simulink model "smm_with_grf_tilting_2d"  (R2014b)
settings: Solver=FixedStepDiscrete  StartTime=0.0  StopTime=inf  FixedStep=sample_time  RelTol=1e-3
undefined symbols (not defined in the file or in its folder): A_lpf_dtau, A_lpf_leg_spring, alpha_apex, alpha_max, alpha_min, B1_lpf_dtau, B1_lpf_leg_spring, B2_lpf_dtau, B2_lpf_leg_spring, boom_mount_angle, boom_pelvis_offset_angle, c_energy, contact_threshold, control_start_time, d_y_boom_com_offset, d_y_boom_hip_offset, d_y_com, desired_torso_angle, dx_avg_desired, enable_torso_wave, fcut_contact, ff_energy_l, ff_energy_r, g, g_reduced, h_boom, HIP_MTR_MAX_CONT_TORQUE, i_robot, initial_com_height, initial_dx, j_leg, j_motor, j_rotor, j_segments, k0_virtual, k_placement, k_sea, kd_lateral, kd_motor, kd_torso, kp_lateral, kp_motor, kp_raibert, kp_torso, l0_leg, l0_min_flight_time, l0_virtual, l0_virtual_raibert, l_boom_projected, l_max, l_retract_delta, l_retract_swing_max, l_retract_swing_min, l_seg, l_yaw_center_to_pelvis, lambda1, lambda2, lateral_offset, lateral_target_angle_left, lateral_target_angle_right ... (+40)
libraries: simulink x24, slrtlib x4, simulink_extras x2
(part 2 of 4)

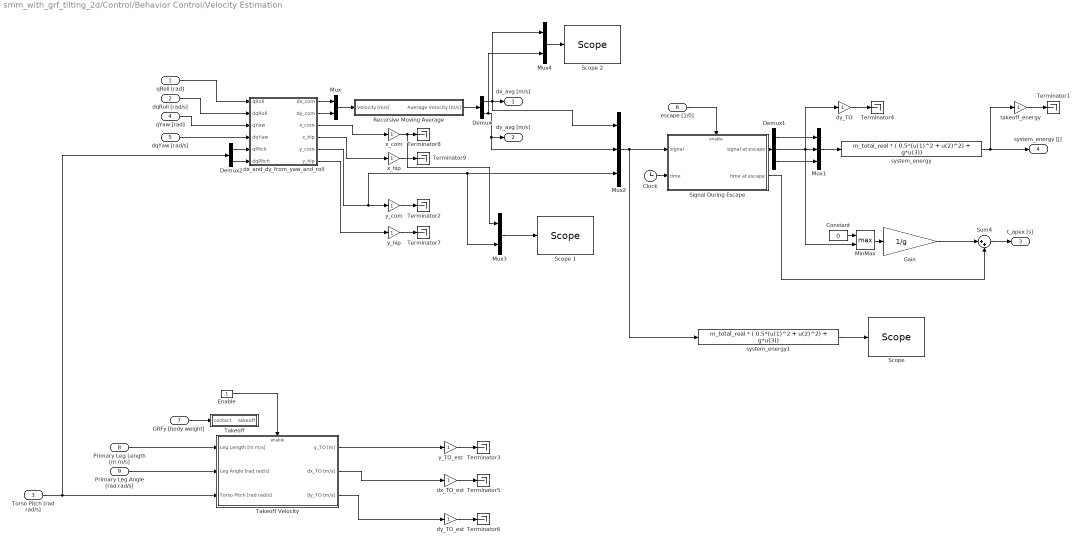
== system smm_with_grf_tilting_2d/Control/Behavior Control/Velocity Estimation ==
  qRoll [rad] : Inport
  dqRoll [rad/s] : Inport  Port=2
  Torso Pitch [rad rad/s] : Inport  Port=3
  qYaw [rad] : Inport  Port=4
  dqYaw [rad/s] : Inport  Port=5
  escape [1/0] : Inport  Port=6
  GRFy [body weight] : Inport  Port=7
  Primary Leg Length [m m/s] : Inport  Port=8
  Primary Leg Angle [rad rad/s] : Inport  Port=9
  Clock : Clock
  Constant : Constant  Value=0
  Demux : Demux  Outputs=2
  Demux1 : Demux  Outputs=3
  Demux2 : Demux  Outputs=2
  Enable : Constant  OutDataTypeStr=boolean
  Gain : Gain  Gain=1/g
  MinMax : MinMax  Function=max  Inputs=2
  Mux : Mux  Inputs=2
  Mux1 : Mux  Inputs=3
  Mux2 : Mux  Inputs=3
  Mux3 : Mux  Inputs=2
  Mux4 : Mux  Inputs=2
  Recursive Moving Average : Subsystem
  "Scope " : slrtlib/Displays and Logging/Scope   scopeno=2  scopetype=Host  autostart=on  viewmode=Graphical redraw  formatstr='%15.6f'  grid=on  ylimits=[0,0]  nosamples=4*250  noprepostsamples=0  interleave=4  triggermode=FreeRun  triggersignal=1  trigsignalfromport=off  triggerlevel=0.0  triggerslope=Either  triggerscope=1  triggersample=0  filename=data.dat  mode=Lazy  writesize=512  autorestart=off  dynamicfilemode=off  maxwritefilesize=512*1024^2
  Scope 1 : slrtlib/Displays and Logging/Scope   scopeno=1  scopetype=Host  autostart=on  viewmode=Graphical redraw  formatstr='%15.6f'  grid=on  ylimits=[0,0]  nosamples=4*250  noprepostsamples=0  interleave=4  triggermode=FreeRun  triggersignal=1  trigsignalfromport=off  triggerlevel=0.0  triggerslope=Either  triggerscope=1  triggersample=0  filename=data.dat  mode=Lazy  writesize=512  autorestart=off  dynamicfilemode=off  maxwritefilesize=512*1024^2
  Scope 2 : slrtlib/Displays and Logging/Scope   scopeno=3  scopetype=Host  autostart=on  viewmode=Graphical redraw  formatstr='%15.6f'  grid=on  ylimits=[0,0]  nosamples=4*250  noprepostsamples=0  interleave=4  triggermode=FreeRun  triggersignal=1  trigsignalfromport=off  triggerlevel=0.0  triggerslope=Either  triggerscope=1  triggersample=0  filename=data.dat  mode=Lazy  writesize=512  autorestart=off  dynamicfilemode=off  maxwritefilesize=512*1024^2
  Signal During Escape : Subsystem
  Sum4 : Sum  Inputs=|++
  Takeoff : Subsystem
  Takeoff Velocity : Subsystem
  Terminator{1..9} (9 alike) : Terminator
  dx_TO_est : Gain
  dx_and_dy_from_yaw_and_roll : MATLAB Function  TreatAsAtomicUnit=on
  dy_TO : Gain
  dy_TO_est : Gain
  system_energy : Fcn  Expr=m_total_real * ( 0.5*(u(1)^2 + u(2)^2) + g*u(3))
  system_energy1 : Fcn  Expr=m_total_real * ( 0.5*(u(1)^2 + u(2)^2) + g*u(3))
  takeoff_energy : Gain
  x_com : Gain
  x_hip : Gain
  y_TO_est : Gain
  y_com : Gain
  y_hip : Gain
  dx_avg [m/s] : Outport
  dy_avg [m/s] : Outport  Port=2
  t_apex [s] : Outport  Port=3
  system_energy [J] : Outport  Port=4
  wires:
  Gain/1 -> Sum4/1
  Enable/1 -> Takeoff Velocity/Enable
  dx_and_dy_from_yaw_and_roll/6(y_hip) -> y_hip/1
  y_hip/1 -> Terminator7/1
  Takeoff Velocity/3(dy_TO [m/s]) -> dy_TO_est/1
  dy_TO_est/1 -> Terminator6/1
  Takeoff Velocity/2(dx_TO [m/s]) -> dx_TO_est/1
  dx_TO_est/1 -> Terminator5/1
  y_TO_est/1 -> Terminator3/1
  Takeoff Velocity/1(y_TO [m]) -> y_TO_est/1
  y_com/1 -> Terminator2/1
  system_energy/1 -> takeoff_energy/1, system_energy [J]/1
  Clock/1 -> Signal During Escape/2(time)
  Demux1/3 -> Mux1/3
  Signal During Escape/2(time at escape) -> Sum4/2
  Signal During Escape/1(signal at escape) -> Demux1/1
  escape [1/0]/1 -> Signal During Escape/Enable
  takeoff_energy/1 -> Terminator1/1
  dy_TO/1 -> Terminator4/1
  Mux1/1 -> system_energy/1
  Demux1/1 -> Mux1/1
  Demux1/2 -> MinMax/2, dy_TO/1, Mux1/2
  Torso Pitch [rad rad/s]/1 -> Demux2/1, Takeoff Velocity/3(Torso Pitch [rad rad/s])
  Primary Leg Angle [rad rad/s]/1 -> Takeoff Velocity/2(Leg Angle [rad rad/s])
  Primary Leg Length [m m/s]/1 -> Takeoff Velocity/1(Leg Length [m m/s])
  Sum4/1 -> t_apex [s]/1
  Demux/2 -> Mux4/2, Mux2/2, dy_avg [m/s]/1
  Demux/1 -> Mux2/1, Mux4/1, dx_avg [m/s]/1
  Mux/1 -> Recursive Moving Average/1(Velocity [m/s])
  dx_and_dy_from_yaw_and_roll/2(dy_com) -> Mux/2
  GRFy [body weight]/1 -> Takeoff/1(contact)
  dx_and_dy_from_yaw_and_roll/1(dx_com) -> Mux/1
  Recursive Moving Average/1(Average Velocity [m/s]) -> Demux/1
  MinMax/1 -> Gain/1
  Constant/1 -> MinMax/1
  x_hip/1 -> Terminator9/1
  x_com/1 -> Mux3/1, Terminator8/1
  dx_and_dy_from_yaw_and_roll/3(x_com) -> x_com/1
  dx_and_dy_from_yaw_and_roll/4(x_hip) -> x_hip/1
  Demux2/1 -> dx_and_dy_from_yaw_and_roll/5(qPitch)
  Demux2/2 -> dx_and_dy_from_yaw_and_roll/6(dqPitch)
  qRoll [rad]/1 -> dx_and_dy_from_yaw_and_roll/1(qRoll)
  dqRoll [rad/s]/1 -> dx_and_dy_from_yaw_and_roll/2(dqRoll)
  qYaw [rad]/1 -> dx_and_dy_from_yaw_and_roll/3(qYaw)
  dqYaw [rad/s]/1 -> dx_and_dy_from_yaw_and_roll/4(dqYaw)
  Mux2/1 -> system_energy1/1, Signal During Escape/1(signal)
  system_energy1/1 -> "Scope "/1
  Mux3/1 -> Scope 1/1
  dx_and_dy_from_yaw_and_roll/5(y_com) -> Mux3/2, Mux2/3, y_com/1
  Mux4/1 -> Scope 2/1

== system smm_with_grf_tilting_2d/Control/Behavior Control/Virtual Spring Calculator ==
  "Stance Leg Angle [rad rad/s] " : Inport
  Stance Leg Length [m m/s] : Inport  Port=2
  Torso Angle [rad rad/s] : Inport  Port=3
  Demux : Demux  Outputs=2
  Demux1 : Demux  Outputs=2
  Demux2 : Demux  Outputs=2
  Mux3 : Mux  Inputs=2
  Mux4 : Mux  Inputs=2
  Virtual Spring Calculations : MATLAB Function  TreatAsAtomicUnit=on
  Spring Length [m m/s] : Outport
  Spring Alpha [rad rad/s] : Outport  Port=2  OutDataTypeStr=double  PortDimensions=2
  wires:
  Stance Leg Length [m m/s]/1 -> Demux1/1
  Mux3/1 -> Spring Length [m m/s]/1
  "Stance Leg Angle [rad rad/s] "/1 -> Demux2/1
  Torso Angle [rad rad/s]/1 -> Demux/1
  Demux/1 -> Virtual Spring Calculations/1(th)
  Demux/2 -> Virtual Spring Calculations/2(dth)
  Demux1/1 -> Virtual Spring Calculations/3(l)
  Demux2/1 -> Virtual Spring Calculations/5(phi)
  Demux2/2 -> Virtual Spring Calculations/6(dphi)
  Demux1/2 -> Virtual Spring Calculations/4(dl)
  Virtual Spring Calculations/1(alpha_v) -> Mux4/1
  Virtual Spring Calculations/2(dalpha_v) -> Mux4/2
  Virtual Spring Calculations/3(l_v) -> Mux3/1
  Virtual Spring Calculations/4(dl_v) -> Mux3/2
  Mux4/1 -> Spring Alpha [rad rad/s]/1

== system smm_with_grf_tilting_2d/Control/Behavior Control/dtau_des ==
  x : Inport
  Gain1 : Gain  Gain=1/sample_time
  difference : simulink/Discrete/Difference  ICPrevInput=0.0  InputProcessing=Inherited  OutMin=[]  OutMax=[]  OutDataType=fixdt(1, 16)  OutScaling=2^-10  DoSatur=off
  two_pole_filter : DiscreteTransferFcn  Numerator=[A_lpf_dtau 0 0]  Denominator=[1 B1_lpf_dtau B2_lpf_dtau]  SampleTime=sample_time
  dx/dt : Outport
  wires:
  two_pole_filter/1 -> dx/dt/1
  x/1 -> Gain1/1
  difference/1 -> two_pole_filter/1
  Gain1/1 -> difference/1

== system smm_with_grf_tilting_2d/Control/Behavior Control/Contact Estimation/Contact Time ==
  Enable : EnablePort  StatesWhenEnabling=reset  ShowOutputPort=on
  Constant : Constant
  Discrete-Time Integrator : DiscreteIntegrator  IntegratorMethod=Accumulation: Forward Euler  gainval=sample_time  ExternalReset=rising  SampleTime=sample_time
  ts [s] : Outport  InitialOutput=[0]
  wires:
  Discrete-Time Integrator/1 -> ts [s]/1
  Enable/1 -> Discrete-Time Integrator/2
  Constant/1 -> Discrete-Time Integrator/1

== system smm_with_grf_tilting_2d/Control/Behavior Control/Contact Estimation/Last Contact Time ==
  ts [s] : Inport
  Trigger : TriggerPort  TriggerType=falling  PortDimensions=1
  Ts [s] : Outport  InitialOutput=[0]
  wires:
  ts [s]/1 -> Ts [s]/1

== system smm_with_grf_tilting_2d/Control/Behavior Control/Contact Estimation/Leg Force Measurements ==
  q : Inport
  w right/left [m m] : Inport  Port=2
  Demux : Demux  Outputs=2
  Divide1 : Product  Inputs=*/
  Divide2 : Product  Inputs=*/
  Spring Stiffness3 : Gain  Gain=k_sea(1)
  Spring Stiffness4 : Gain  Gain=k_sea(3)
  Spring Stiffness5 : Gain  Gain=k_sea(2)
  Spring Stiffness6 : Gain  Gain=k_sea(4)
  Sum{1..6} (6 alike) : Sum  Inputs=-+|
  backGearL : Selector  InputPortWidth=13  Indices=[6]
  backGearR : Selector  InputPortWidth=13  Indices=[2]
  backJointL : Selector  InputPortWidth=13  Indices=[5]
  backJointR : Selector  InputPortWidth=13  Indices=[1]
  frontGearL : Selector  InputPortWidth=13  Indices=[8]
  frontGearR : Selector  InputPortWidth=13  Indices=[4]
  frontJointL : Selector  InputPortWidth=13  Indices=[7]
  frontJointR : Selector  InputPortWidth=13  Indices=[3]
  Right Leg Force [N] : Outport
  Left Leg Force [N] : Outport  Port=2
  wires:
  Sum3/1 -> Spring Stiffness6/1
  Sum2/1 -> Spring Stiffness4/1
  backJointL/1 -> Sum2/1
  frontGearL/1 -> Sum3/2
  frontJointL/1 -> Sum3/1
  backGearL/1 -> Sum2/2
  Sum6/1 -> Spring Stiffness3/1
  Sum1/1 -> Spring Stiffness5/1
  backJointR/1 -> Sum6/1
  frontGearR/1 -> Sum1/2
  frontJointR/1 -> Sum1/1
  backGearR/1 -> Sum6/2
  q/1 -> backGearR/1, backJointL/1, backGearL/1, frontJointR/1, frontGearR/1, frontJointL/1, frontGearL/1, backJointR/1
  Spring Stiffness3/1 -> Sum4/1
  Spring Stiffness5/1 -> Sum4/2
  Spring Stiffness6/1 -> Sum5/2
  Spring Stiffness4/1 -> Sum5/1
  Sum4/1 -> Divide1/1
  Sum5/1 -> Divide2/1
  w right/left [m m]/1 -> Demux/1
  Demux/1 -> Divide1/2
  Demux/2 -> Divide2/2
  Divide1/1 -> Right Leg Force [N]/1
  Divide2/1 -> Left Leg Force [N]/1

== system smm_with_grf_tilting_2d/Control/Behavior Control/Contact Estimation/Vertical Spring Force ==
  theta [rad] : Inport
  phi [rad] : Inport  Port=2
  Force [N] : Inport  Port=3
  Gain : Gain  Gain=-1
  Product : Product
  Sum : Sum  Inputs=++|
  Trigonometric Function : Trigonometry  Operator=cos
  Vertical Force [N] : Outport
  wires:
  Gain/1 -> Vertical Force [N]/1
  Sum/1 -> Trigonometric Function/1
  Product/1 -> Gain/1
  Trigonometric Function/1 -> Product/2
  theta [rad]/1 -> Sum/1
  phi [rad]/1 -> Sum/2
  Force [N]/1 -> Product/1

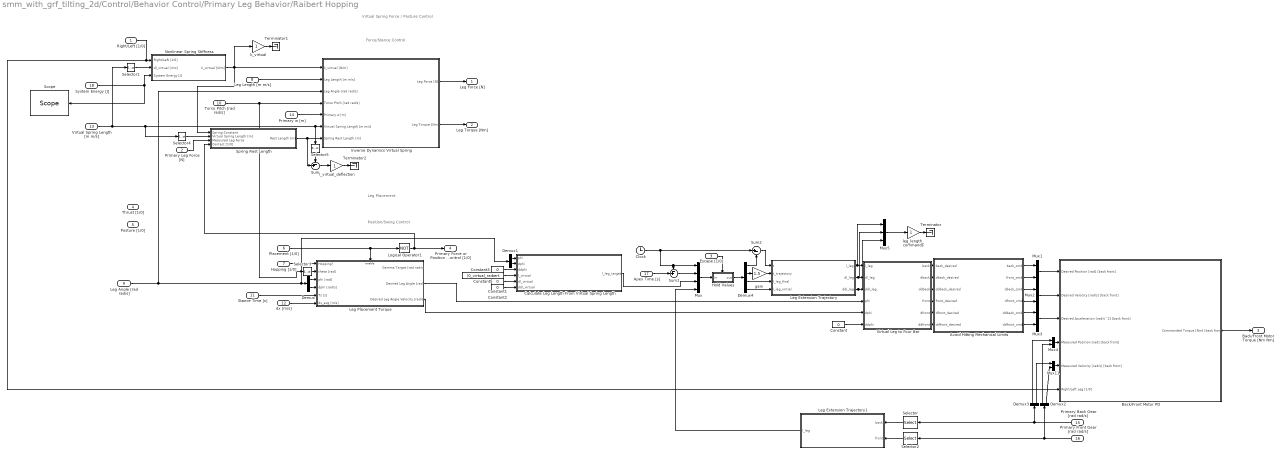
== system smm_with_grf_tilting_2d/Control/Behavior Control/Primary Leg Behavior/Raibert Hopping ==
  note: Leg Placement
  note: Virtual Spring Force / Posture Control
  note: Force/Stance Control
  note: Position/Swing Control
  Right/Left [1/0] : Inport
  Primary Leg Force [N] : Inport  Port=2
  Escape [1/0] : Inport  Port=3
  Thrust [1/0] : Inport  Port=4
  Posture [1/0] : Inport  Port=5
  Placement [1/0] : Inport  Port=6
  Hopping [1/0] : Inport  Port=7
  Leg Length [m m/s] : Inport  Port=8
  Leg Angle [rad rad/s] : Inport  Port=9
  Torso Pitch [rad rad/s] : Inport  Port=10
  Stance Time [s] : Inport  Port=11
  dx [m/s] : Inport  Port=12
  Virtual Spring Length [m m/s] : Inport  Port=13
  Primary w [m] : Inport  Port=14
  Primary Back Gear [rad rad/s] : Inport  Port=15
  Primary Front Gear [rad rad/s] : Inport  Port=16
  Apex Time [s] : Inport  Port=17
  System Energy [J] : Inport  Port=18
  Avoid Hitting Mechanical Limits : MATLAB Function  TreatAsAtomicUnit=on
  Back/Front Motor PD : Subsystem
  Calculate Leg Length From Virtual Spring Length : MATLAB Function  TreatAsAtomicUnit=on
  Clock : Clock
  Constant{,1..3} (4 alike) : Constant  Value=0
  Constant5 : Constant  Value=l0_virtual_raibert
  Demux{,1..3} (4 alike) : Demux  Outputs=2
  Demux4 : Demux
  Hold Values : Subsystem
  Inverse Dynamics Virtual Spring : Subsystem
  Leg Extension Trajectory : MATLAB Function  TreatAsAtomicUnit=on
  Leg Extension Trajectory1 : MATLAB Function  TreatAsAtomicUnit=on
  Leg Placement Torque : Subsystem
  Logical Operator1 : Logic  Operator=NOT  AllPortsSameDT=off  OutDataTypeStr=boolean
  Mux : Mux
  Mux{1..4,11} (5 alike) : Mux  Inputs=2
  Mux5 : Mux  Inputs=3
  Nonlinear Spring Stiffness : Subsystem
  "Scope " : slrtlib/Displays and Logging/Scope   scopeno=5  scopetype=Host  autostart=on  viewmode=Graphical redraw  formatstr='%15.6f'  grid=on  ylimits=[0,0]  nosamples=4*250  noprepostsamples=0  interleave=4  triggermode=FreeRun  triggersignal=1  trigsignalfromport=off  triggerlevel=0.0  triggerslope=Either  triggerscope=1  triggersample=0  filename=data.dat  mode=Lazy  writesize=512  autorestart=off  dynamicfilemode=off  maxwritefilesize=512*1024^2
  Selector{,2..5} (5 alike) : Selector  InputPortWidth=2  Indices=[1]
  Selector1 : Selector  InputPortWidth=2  Indices=[2]
  Spring Rest Length : Subsystem
  Sum : Sum  Inputs=-+|
  Sum1 : Sum  Inputs=-+|
  Sum2 : Sum  Inputs=|+-
  Terminator : Terminator
  Terminator1 : Terminator
  Terminator2 : Terminator
  Virtual Leg to Four Bar : MATLAB Function  TreatAsAtomicUnit=on
  gain : Gain  Gain=1.5
  k_virtual : Gain
  l_virtual_deflection : Gain
  leg_length_commands : Gain
  Leg Force [N] : Outport
  Leg Torque [Nm] : Outport  Port=2
  Back/Front Motor Torque [Nm Nm] : Outport  Port=3
  Primary Force or Position Control [1/0] : Outport  Port=4  OutDataTypeStr=boolean
  wires:
  Nonlinear Spring Stiffness/1(k_virtual [N/m]) -> Spring Rest Length/1(Spring Constant), k_virtual/1, Inverse Dynamics Virtual Spring/1(k_virtual [N/m])
  Selector1/1 -> Nonlinear Spring Stiffness/2(dl_virtual [m/s])
  Demux/1 -> Leg Placement Torque/3(phi [rad])
  Demux/2 -> Leg Placement Torque/4(dphi [rad/s])
  Hopping [1/0]/1 -> Leg Placement Torque/1(Hopping?)
  Placement [1/0]/1 -> Leg Placement Torque/Enable, Logical Operator1/1
  Selector3/1 -> Leg Placement Torque/2(theta [rad])
  Torso Pitch [rad rad/s]/1 -> Selector3/1, Inverse Dynamics Virtual Spring/4(Torso Pitch [rad rad/s])
  Leg Length [m m/s]/1 -> Inverse Dynamics Virtual Spring/2(Leg Length [m m/s])
  dx [m/s]/1 -> Leg Placement Torque/6(dx_avg [m/s])
  Stance Time [s]/1 -> Leg Placement Torque/5(Ts [s])
  Virtual Spring Length [m m/s]/1 -> Inverse Dynamics Virtual Spring/6(Virtual Spring Length [m m/s]), Selector5/1, Selector4/1, Selector1/1
  Leg Angle [rad rad/s]/1 -> Demux1/1, Demux/1, Inverse Dynamics Virtual Spring/3(Leg Angle [rad rad/s])
  Primary w [m]/1 -> Inverse Dynamics Virtual Spring/5(Primary w [m])
  Inverse Dynamics Virtual Spring/2(Leg Torque [Nm]) -> Leg Torque [Nm]/1
  Inverse Dynamics Virtual Spring/1(Leg Force [N]) -> Leg Force [N]/1
  Virtual Leg to Four Bar/1(back) -> Avoid Hitting Mechanical Limits/1(back_desired)
  Virtual Leg to Four Bar/2(dback) -> Avoid Hitting Mechanical Limits/2(dback_desired)
  Virtual Leg to Four Bar/3(ddback) -> Avoid Hitting Mechanical Limits/3(ddback_desired)
  Virtual Leg to Four Bar/4(front) -> Avoid Hitting Mechanical Limits/4(front_desired)
  Virtual Leg to Four Bar/5(dfront) -> Avoid Hitting Mechanical Limits/5(dfront_desired)
  Virtual Leg to Four Bar/6(ddfront) -> Avoid Hitting Mechanical Limits/6(ddfront_desired)
  Mux11/1 -> Back/Front Motor PD/5(Measured Velocity [rad/s] [back front])
  Demux2/2 -> Mux11/2
  Mux4/1 -> Back/Front Motor PD/4(Measured Position [rad] [back front])
  Mux1/1 -> Back/Front Motor PD/1(Desired Position [rad] [back front])
  Demux3/2 -> Mux11/1
  Demux3/1 -> Mux4/1
  Avoid Hitting Mechanical Limits/2(front_cmd) -> Mux1/2
  Avoid Hitting Mechanical Limits/1(back_cmd) -> Mux1/1
  Demux2/1 -> Mux4/2
  Avoid Hitting Mechanical Limits/3(dback_cmd) -> Mux2/1
  Avoid Hitting Mechanical Limits/4(dfront_cmd) -> Mux2/2
  Avoid Hitting Mechanical Limits/5(ddback_cmd) -> Mux3/1
  Avoid Hitting Mechanical Limits/6(ddfront_cmd) -> Mux3/2
  Mux2/1 -> Back/Front Motor PD/2(Desired Velocity [rad/s] [back front])
  Mux3/1 -> Back/Front Motor PD/3(Desired Acceleration [rad/s^2] [back front])
  Logical Operator1/1 -> Spring Rest Length/4(Contact [1/0]), Primary Force or Position Control [1/0]/1
  Back/Front Motor PD/1(Commanded Torque [Nm] [back front]) -> Back/Front Motor Torque [Nm Nm]/1
  Primary Back Gear [rad rad/s]/1 -> Demux3/1, Selector/1
  Primary Front Gear [rad rad/s]/1 -> Selector2/1, Demux2/1
  Constant/1 -> Virtual Leg to Four Bar/6(ddphi)
  Leg Placement Torque/2(Desired Leg Angle [rad]) -> Virtual Leg to Four Bar/4(phi)
  Leg Placement Torque/3(Desired Leg Angle Velocity [rad/s]) -> Virtual Leg to Four Bar/5(dphi)
  Constant5/1 -> Calculate Leg Length From Virtual Spring Length/4(l_virtual)
  Constant1/1 -> Calculate Leg Length From Virtual Spring Length/5(dl_virtual)
  Constant2/1 -> Calculate Leg Length From Virtual Spring Length/6(ddl_virtual)
  Constant3/1 -> Calculate Leg Length From Virtual Spring Length/3(ddphi)
  Demux1/1 -> Calculate Leg Length From Virtual Spring Length/1(phi)
  Demux1/2 -> Calculate Leg Length From Virtual Spring Length/2(dphi)
  Leg Extension Trajectory/1(l_leg) -> Mux5/1, Virtual Leg to Four Bar/1(l_leg)
  Leg Extension Trajectory/3(ddl_leg) -> Mux5/3, Virtual Leg to Four Bar/3(ddl_leg)
  Apex Time [s]/1 -> Sum1/2
  Clock/1 -> Sum1/1, Mux/1, Sum2/1
  Sum2/1 -> Leg Extension Trajectory/1(t)
  Mux5/1 -> leg_length_commands/1
  Leg Extension Trajectory/2(dl_leg) -> Mux5/2, Virtual Leg to Four Bar/2(dl_leg)
  leg_length_commands/1 -> Terminator/1
  Demux4/2 -> gain/1
  Sum1/1 -> Mux/2
  Calculate Leg Length From Virtual Spring Length/1(l_leg_target) -> Mux/3
  Demux4/4 -> Leg Extension Trajectory/4(l_leg_initial)
  Demux4/3 -> Leg Extension Trajectory/3(l_leg_final)
  Demux4/1 -> Sum2/2
  Selector/1 -> Leg Extension Trajectory1/1(back)
  Selector2/1 -> Leg Extension Trajectory1/2(front)
  Right/Left [1/0]/1 -> Back/Front Motor PD/6(Right/Left Leg [1/0]), Nonlinear Spring Stiffness/1(Right/Left [1/0])
  Hold Values/1(out) -> Demux4/1
  Mux/1 -> Hold Values/1(in)
  gain/1 -> Leg Extension Trajectory/2(t_trajectory)
  Escape [1/0]/1 -> Hold Values/Trigger
  Leg Extension Trajectory1/1(l_leg) -> Mux/4
  k_virtual/1 -> Terminator1/1
  l_virtual_deflection/1 -> Terminator2/1
  Sum/1 -> l_virtual_deflection/1
  Selector5/1 -> Sum/1
  Spring Rest Length/1(Rest Length [m]) -> Sum/2, Inverse Dynamics Virtual Spring/7(Spring Rest Length [m])
  Selector4/1 -> Spring Rest Length/2(Virtual Spring Length [m])
  Primary Leg Force [N]/1 -> Spring Rest Length/3(Measured Leg Force)
  System Energy [J]/1 -> Nonlinear Spring Stiffness/3(System Energy [J]), "Scope "/1

== system smm_with_grf_tilting_2d/Control/Behavior Control/Primary Leg Behavior/SMM 01 ==
  note: Stance
  note: Swing
  Right/Left [1/0] : Inport
  Escape [1/0] : Inport  Port=2
  Posture [1/0] : Inport  Port=3
  Placement [1/0] : Inport  Port=4
  Primary Leg Angle [rad rad/s] : Inport  Port=5
  Primary Leg Length [m m/s] : Inport  Port=6
  Torso Pitch [rad rad/s] : Inport  Port=7
  Virtual Spring Length [m m/s] : Inport  Port=8
  Apex Time [s] : Inport  Port=9
  System Energy [J] : Inport  Port=10
  Primary Back Gear [rad rad/s] : Inport  Port=11
  Primary Front Gear [rad rad/s] : Inport  Port=12
  Primary w [m] : Inport  Port=13
  Logical Operator : Logic  Operator=NOT  AllPortsSameDT=off  OutDataTypeStr=boolean
  Primary Stance Phase : Subsystem
  Primary Swing Phase : Subsystem
  Leg Force [Nm] : Outport
  Leg Torque [Nm] : Outport  Port=2
  Back/Front Motor Torque [Nm Nm] : Outport  Port=3
  Primary Force or Position Control [1/0] : Outport  Port=4  OutDataTypeStr=boolean
  wires:
  Primary w [m]/1 -> Primary Stance Phase/7(Primary w [m])
  Logical Operator/1 -> Primary Force or Position Control [1/0]/1
  Primary Stance Phase/2(Leg Force Command [Nm]) -> Leg Force [Nm]/1
  Primary Stance Phase/1(Leg Torque Command [Nm]) -> Leg Torque [Nm]/1
  Escape [1/0]/1 -> Primary Swing Phase/1(Escape [1/0])
  Virtual Spring Length [m m/s]/1 -> Primary Stance Phase/6(Virtual Spring Length [m m/s])
  System Energy [J]/1 -> Primary Stance Phase/5(System Energy [J])
  Posture [1/0]/1 -> Primary Stance Phase/3(Enable Posture Control [1/0])
  Primary Leg Angle [rad rad/s]/1 -> Primary Swing Phase/3(Primary Leg Angle [rad rad/s]), Primary Stance Phase/8(Primary Leg Angle [rad rad/s])
  Primary Swing Phase/1(Back/Front Motor Torque Command [Nm Nm]) -> Back/Front Motor Torque [Nm Nm]/1
  Primary Front Gear [rad rad/s]/1 -> Primary Swing Phase/7(Primary Front Gear [rad rad/s])
  Primary Back Gear [rad rad/s]/1 -> Primary Swing Phase/6(Primary Back Gear [rad rad/s])
  Apex Time [s]/1 -> Primary Swing Phase/5(Time of Apex [s])
  Placement [1/0]/1 -> Logical Operator/1
  Right/Left [1/0]/1 -> Primary Stance Phase/4(Right/Left Primary [1/0]), Primary Swing Phase/8(Right/Left Primary [1/0])
  Primary Leg Length [m m/s]/1 -> Primary Swing Phase/2(Primary Leg Length [m m/s]), Primary Stance Phase/1(Primary Leg Length [m m/s])
  Torso Pitch [rad rad/s]/1 -> Primary Swing Phase/4(Torso Pitch [rad rad/s]), Primary Stance Phase/2(Torso Pitch [rad rad/s])

== system smm_with_grf_tilting_2d/Control/Behavior Control/Secondary Leg Behavior/Back//Front Motor PD ==
  Desired Position [rad] [back front] : Inport
  Desired Velocity [rad/s] [back front] : Inport  Port=2
  Desired Acceleration [rad/s^2] [back front] : Inport  Port=3
  Measured Position [rad] [back front] : Inport  Port=4
  Measured Velocity [rad/s] [back front] : Inport  Port=5
  Right/Left Leg [1/0] : Inport  Port=6
  Friction Compensation : Subsystem
  Product : Product
  Sum1 : Sum  Inputs=|++
  Sum2 : Sum  Inputs=|++
  Sum7 : Sum  Inputs=|+-
  Sum8 : Sum  Inputs=|+-
  Sum9 : Sum
  Switch : Switch  Criteria=u2 ~= 0
  kd : Gain  Gain=kd_motor
  kp : Gain  Gain=kp_motor
  left_inertias : Constant  Value=j_segments(3:4)
  reflected inertia : Constant  Value=j_motor
  right_inertias : Constant  Value=j_segments(1:2)
  Commanded Torque [Nm] [back front] : Outport
  wires:
  kp/1 -> Sum9/1
  Sum7/1 -> kp/1
  Measured Position [rad] [back front]/1 -> Sum7/2
  Sum9/1 -> Sum1/1
  Sum8/1 -> kd/1
  Desired Position [rad] [back front]/1 -> Sum7/1
  kd/1 -> Sum9/2
  Measured Velocity [rad/s] [back front]/1 -> Sum8/2
  Sum1/1 -> Sum2/1
  Desired Acceleration [rad/s^2] [back front]/1 -> Product/1
  Product/1 -> Sum1/2
  Right/Left Leg [1/0]/1 -> Friction Compensation/1(Right/Left [1/0]), Switch/2
  right_inertias/1 -> Switch/1
  left_inertias/1 -> Switch/3
  Sum2/1 -> Commanded Torque [Nm] [back front]/1
  Desired Velocity [rad/s] [back front]/1 -> Friction Compensation/2(Commanded Velocity [rad/s] [back front]), Sum8/1
  reflected inertia/1 -> Product/2

== system smm_with_grf_tilting_2d/Control/Behavior Control/Velocity Estimation/Recursive Moving Average ==
  Velocity [m/s] : Inport
  Delay : Delay  DelayLength=velocity_avg_samples  InitialCondition=0  UseCircularBuffer=on  SampleTime=sample_time
  Gain : Gain  Gain=1/velocity_avg_samples
  Sum : Sum  Inputs=-++
  Unit Delay : UnitDelay  SampleTime=sample_time
  Average Velocity [m/s] : Outport
  wires:
  Unit Delay/1 -> Sum/3
  Gain/1 -> Average Velocity [m/s]/1
  Delay/1 -> Sum/1
  Sum/1 -> Gain/1, Unit Delay/1
  Velocity [m/s]/1 -> Sum/2, Delay/1

== system smm_with_grf_tilting_2d/Control/Behavior Control/Velocity Estimation/Signal During Escape ==
  signal : Inport
  time : Inport  Port=2
  Enable : EnablePort
  signal at escape : Outport  InitialOutput=[0 0 y_com_desired-0.1182]
  time at escape : Outport  Port=2
  wires:
  time/1 -> time at escape/1
  signal/1 -> signal at escape/1

== system smm_with_grf_tilting_2d/Control/Behavior Control/Velocity Estimation/Takeoff ==
  contact : Inport
  Compare To Constant : simulink/Logic and Bit Operations/Compare To Constant  relop=<=  const=TO_threshold  OutDataTypeStr=boolean
  Compare To Constant1 : simulink/Logic and Bit Operations/Compare To Constant  relop=>  const=TO_threshold  OutDataTypeStr=boolean
  Logical Operator : Logic  AllPortsSameDT=off  OutDataTypeStr=boolean
  Unit Delay1 : UnitDelay  SampleTime=sample_time
  takeoff : Outport
  wires:
  Unit Delay1/1 -> Compare To Constant1/1
  Logical Operator/1 -> takeoff/1
  contact/1 -> Unit Delay1/1, Compare To Constant/1
  Compare To Constant/1 -> Logical Operator/2
  Compare To Constant1/1 -> Logical Operator/1

== system smm_with_grf_tilting_2d/Control/Behavior Control/Velocity Estimation/Takeoff Velocity ==
  Leg Length [m m/s] : Inport
  Leg Angle [rad rad/s] : Inport  Port=2
  Torso Pitch [rad rad/s] : Inport  Port=3
  Enable : EnablePort
  Demux2 : Demux  Outputs=2
  Demux3 : Demux  Outputs=2
  Demux4 : Demux  Outputs=2
  vertical_velocity : MATLAB Function  TreatAsAtomicUnit=on
  y_TO [m] : Outport  InitialOutput=[initial_com_height]
  dx_TO [m/s] : Outport  Port=2  InitialOutput=[initial_dx]
  dy_TO [m/s] : Outport  Port=3  InitialOutput=[0]
  wires:
  vertical_velocity/3(dy) -> dy_TO [m/s]/1
  vertical_velocity/2(dx) -> dx_TO [m/s]/1
  vertical_velocity/1(y) -> y_TO [m]/1
  Demux2/2 -> vertical_velocity/2(dl)
  Demux4/2 -> vertical_velocity/6(dqPitch)
  Leg Angle [rad rad/s]/1 -> Demux3/1
  Demux3/1 -> vertical_velocity/3(phi)
  Demux3/2 -> vertical_velocity/4(dphi)
  Torso Pitch [rad rad/s]/1 -> Demux4/1
  Demux4/1 -> vertical_velocity/5(qPitch)
  Leg Length [m m/s]/1 -> Demux2/1
  Demux2/1 -> vertical_velocity/1(l)

== system smm_with_grf_tilting_2d/Control/Behavior Control/Primary Leg Behavior/Raibert Hopping/Back//Front Motor PD ==
  Desired Position [rad] [back front] : Inport
  Desired Velocity [rad/s] [back front] : Inport  Port=2
  Desired Acceleration [rad/s^2] [back front] : Inport  Port=3
  Measured Position [rad] [back front] : Inport  Port=4
  Measured Velocity [rad/s] [back front] : Inport  Port=5
  Right/Left Leg [1/0] : Inport  Port=6
  Friction Compensation : Subsystem
  Product : Product
  Sum1 : Sum  Inputs=|++
  Sum2 : Sum  Inputs=|++
  Sum7 : Sum  Inputs=|+-
  Sum8 : Sum  Inputs=|+-
  Sum9 : Sum
  kd : Gain  Gain=kd_motor
  kp : Gain  Gain=kp_motor
  reflected inertia : Constant  Value=j_motor
  Commanded Torque [Nm] [back front] : Outport
  wires:
  kp/1 -> Sum9/1
  Sum7/1 -> kp/1
  Measured Position [rad] [back front]/1 -> Sum7/2
  Sum9/1 -> Sum1/1
  Sum8/1 -> kd/1
  Desired Position [rad] [back front]/1 -> Sum7/1
  kd/1 -> Sum9/2
  Measured Velocity [rad/s] [back front]/1 -> Sum8/2
  Sum1/1 -> Sum2/1
  Desired Acceleration [rad/s^2] [back front]/1 -> Product/1
  Product/1 -> Sum1/2
  Right/Left Leg [1/0]/1 -> Friction Compensation/1(Right/Left [1/0])
  Sum2/1 -> Commanded Torque [Nm] [back front]/1
  Desired Velocity [rad/s] [back front]/1 -> Friction Compensation/2(Commanded Velocity [rad/s] [back front]), Sum8/1
  reflected inertia/1 -> Product/2
  Friction Compensation/1(Friction Compensation [Nm]) -> Sum2/2

== system smm_with_grf_tilting_2d/Control/Behavior Control/Primary Leg Behavior/Raibert Hopping/Hold Values ==
  in : Inport
  Trigger : TriggerPort  ShowOutputPort=on  PortDimensions=1
  Subsystem : Subsystem
  out : Outport
  wires:
  in/1 -> Subsystem/1(in)
  Subsystem/1(out) -> out/1
  Trigger/1 -> Subsystem/Enable

== system smm_with_grf_tilting_2d/Control/Behavior Control/Primary Leg Behavior/Raibert Hopping/Inverse Dynamics Virtual Spring ==
  k_virtual [N/m] : Inport
  Leg Length [m m/s] : Inport  Port=2
  Leg Angle [rad rad/s] : Inport  Port=3
  Torso Pitch [rad rad/s] : Inport  Port=4
  Primary w [m] : Inport  Port=5
  Virtual Spring Length [m m/s] : Inport  Port=6
  Spring Rest Length [m] : Inport  Port=7
  Angle Sine Wave : Subsystem  Commented=on
  Constant1 : Constant  Commented=on  Value=enable_torso_wave
  Constant2 : Constant  Value=0
  Constant3 : Constant  Value=desired_torso_angle
  Demux5 : Demux  Outputs=2
  GRF_angle : Gain
  GRFx_target : Gain
  GRFy_target : Gain
  Leg Force-Torque Distribution : Subsystem
  Spring Torques : Selector  InputPortWidth=7  Indices=[6 7]
  Terminator : Terminator
  Terminator1 : Terminator
  Terminator2 : Terminator
  target_GRF_inverse_dynamics : MATLAB Function  TreatAsAtomicUnit=on
  Leg Force [N] : Outport
  Leg Torque [Nm] : Outport  Port=2
  wires:
  Leg Force-Torque Distribution/1(Leg Force [N]) -> Leg Force [N]/1
  GRF_angle/1 -> Terminator2/1
  GRFy_target/1 -> Terminator1/1
  GRFx_target/1 -> Terminator/1
  Leg Angle [rad rad/s]/1 -> target_GRF_inverse_dynamics/4(phi)
  Torso Pitch [rad rad/s]/1 -> target_GRF_inverse_dynamics/3(theta)
  target_GRF_inverse_dynamics/4(GRF_angle) -> GRF_angle/1
  target_GRF_inverse_dynamics/3(GRFy) -> GRFy_target/1
  target_GRF_inverse_dynamics/2(GRFx) -> GRFx_target/1
  Leg Force-Torque Distribution/2(Leg Torque [Nm]) -> Leg Torque [Nm]/1
  Primary w [m]/1 -> target_GRF_inverse_dynamics/6(w), Leg Force-Torque Distribution/3(w [m])
  Spring Torques/1 -> Demux5/1
  Demux5/1 -> Leg Force-Torque Distribution/1(Front Spring Torque [Nm])
  Demux5/2 -> Leg Force-Torque Distribution/2(Back Spring Torque [Nm])
  target_GRF_inverse_dynamics/1(z) -> Spring Torques/1
  Constant2/1 -> target_GRF_inverse_dynamics/8(tau_rotor_b), target_GRF_inverse_dynamics/7(tau_rotor_f)
  Leg Length [m m/s]/1 -> target_GRF_inverse_dynamics/5(l_leg)
  k_virtual [N/m]/1 -> target_GRF_inverse_dynamics/1(k_virtual)
  Virtual Spring Length [m m/s]/1 -> target_GRF_inverse_dynamics/2(l_virtual)
  Constant1/1 -> Angle Sine Wave/Enable
  Spring Rest Length [m]/1 -> target_GRF_inverse_dynamics/9(l_virtual_rest)
  Constant3/1 -> target_GRF_inverse_dynamics/10(desired_torso_angle)

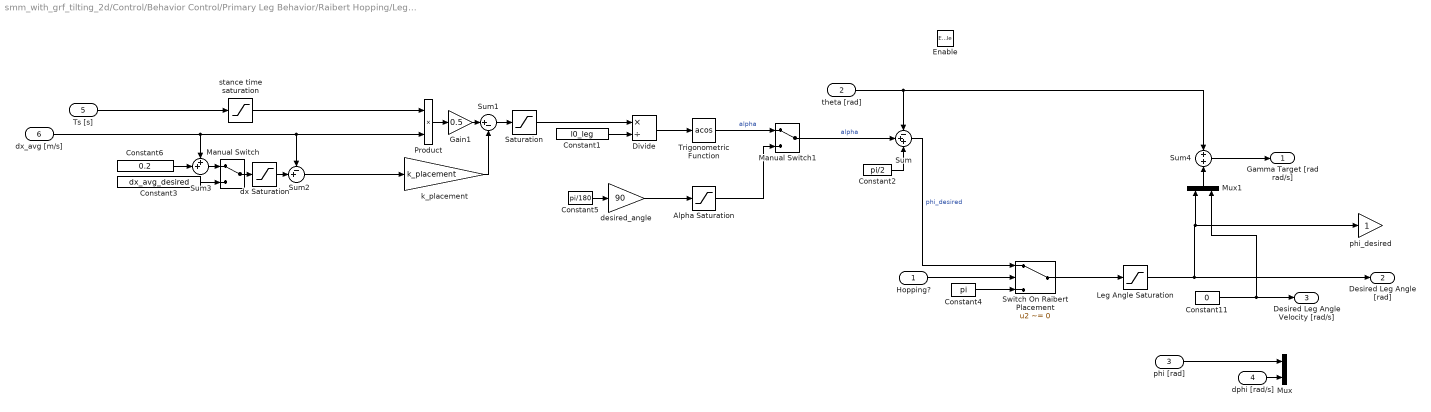
== system smm_with_grf_tilting_2d/Control/Behavior Control/Primary Leg Behavior/Raibert Hopping/Leg Placement Torque ==
  Hopping? : Inport
  theta [rad] : Inport  Port=2
  phi [rad] : Inport  Port=3
  dphi [rad/s] : Inport  Port=4
  Ts [s] : Inport  Port=5
  dx_avg [m/s] : Inport  Port=6
  Enable : EnablePort  StatesWhenEnabling=reset
  Alpha Saturation : Saturate  UpperLimit=alpha_max  LowerLimit=alpha_min
      settings: AttributesFormatString=Hi: %<UpperLimit>\nLo: %<LowerLimit>
  Constant1 : Constant  Value=l0_leg
  Constant11 : Constant  Value=0
  Constant2 : Constant  Value=pi/2
  Constant3 : Constant  Value=dx_avg_desired
  Constant4 : Constant  Value=pi
  Constant5 : Constant  Value=pi/180
  Constant6 : Constant  Value=0.2
  Divide : Product  Inputs=*/
  Gain1 : Gain  Gain=0.5
  Leg Angle Saturation : Saturate  UpperLimit=max_leg_angle  LowerLimit=min_leg_angle
      settings: AttributesFormatString=Hi: %<UpperLimit>\nLo: %<LowerLimit>
  Manual Switch : ManualSwitch
  Manual Switch1 : ManualSwitch
  Mux : Mux  Inputs=2
  Mux1 : Mux  Inputs=2
  Product : Product
  Saturation : Saturate  UpperLimit=x_limit  LowerLimit=-x_limit
      settings: AttributesFormatString=Hi: %<UpperLimit>\nLo: %<LowerLimit>
  Sum : Sum  Inputs=-++
  Sum1 : Sum  Inputs=|+-
  Sum2 : Sum  Inputs=-+|
  Sum3 : Sum  Inputs=++|
  Sum4 : Sum  Inputs=+|+
  Switch On Raibert Placement : Switch  Criteria=u2 ~= 0
  Trigonometric Function : Trigonometry  Operator=acos
  desired_angle : Gain  Gain=90
  dx Saturation : Saturate  UpperLimit=dx_avg_desired  LowerLimit=0
      settings: AttributesFormatString=Hi: %<UpperLimit>\nLo: %<LowerLimit>
  k_placement : Gain  Gain=k_placement
  phi_desired : Gain
  stance time saturation : Saturate  UpperLimit=1  LowerLimit=0
      settings: AttributesFormatString=Hi: %<UpperLimit>\nLo: %<LowerLimit>
  Gamma Target [rad rad/s] : Outport  OutputWhenDisabled=reset  InitialOutput=[0]
  Desired Leg Angle [rad] : Outport  Port=2  OutputWhenDisabled=reset  InitialOutput=[0]
  Desired Leg Angle Velocity [rad/s] : Outport  Port=3  OutputWhenDisabled=reset  InitialOutput=[0]
  wires:
  desired_angle/1 -> Alpha Saturation/1
  Alpha Saturation/1 -> Manual Switch1/2
  Sum2/1 -> k_placement/1
  Trigonometric Function/1 -> Manual Switch1/1  "alpha"
  Mux1/1 -> Sum4/2
  Sum4/1 -> Gamma Target [rad rad/s]/1
  Constant11/1 -> Desired Leg Angle Velocity [rad/s]/1, Mux1/2
  phi [rad]/1 -> Mux/1
  dphi [rad/s]/1 -> Mux/2
  Ts [s]/1 -> stance time saturation/1
  Product/1 -> Gain1/1
  Gain1/1 -> Sum1/1
  Saturation/1 -> Divide/1
  Constant1/1 -> Divide/2
  Divide/1 -> Trigonometric Function/1
  Manual Switch1/1 -> Sum/2  "alpha"
  Constant2/1 -> Sum/3
  theta [rad]/1 -> Sum4/1, Sum/1
  Sum/1 -> Switch On Raibert Placement/1  "phi_desired"
  Sum1/1 -> Saturation/1
  k_placement/1 -> Sum1/2
  dx Saturation/1 -> Sum2/2
  Constant4/1 -> Switch On Raibert Placement/3
  Hopping?/1 -> Switch On Raibert Placement/2
  Leg Angle Saturation/1 -> Desired Leg Angle [rad]/1, Mux1/1, phi_desired/1
  Constant5/1 -> desired_angle/1
  Switch On Raibert Placement/1 -> Leg Angle Saturation/1
  Manual Switch/1 -> dx Saturation/1
  Constant3/1 -> Manual Switch/2
  dx_avg [m/s]/1 -> Sum3/1, Sum2/1, Product/2
  Constant6/1 -> Sum3/2
  Sum3/1 -> Manual Switch/1
  stance time saturation/1 -> Product/1

== system smm_with_grf_tilting_2d/Control/Behavior Control/Primary Leg Behavior/Raibert Hopping/Nonlinear Spring Stiffness ==
  Right/Left [1/0] : Inport
  dl_virtual [m/s] : Inport  Port=2
  System Energy [J] : Inport  Port=3
  E_target1 : Constant  Value=ff_energy_r
  E_target2 : Constant  Value=ff_energy_l
  Product : Product  Inputs=3
  Saturation : Saturate  UpperLimit=max_kp_raibert  LowerLimit=min_kp_raibert  ZeroCross=off
  Sum : Sum  Inputs=+|-
  Sum1 : Sum  Inputs=+-|
  Sum2 : Sum  Inputs=--|
  Switch1 : Switch  Criteria=u2 ~= 0
  c_energy : Constant  Value=c_energy
  c_energy1 : Constant  Value=raibert_target_energy
  k0_virtual : Constant  Value=kp_raibert
  k_virtual [N/m] : Outport
  wires:
  Sum2/1 -> Product/1
  c_energy1/1 -> Sum1/1
  Switch1/1 -> Sum2/2
  Right/Left [1/0]/1 -> Switch1/2
  E_target2/1 -> Switch1/3
  E_target1/1 -> Switch1/1
  dl_virtual [m/s]/1 -> Product/2
  c_energy/1 -> Product/3
  k0_virtual/1 -> Sum/1
  Saturation/1 -> k_virtual [N/m]/1
  Sum/1 -> Saturation/1
  Product/1 -> Sum/2
  System Energy [J]/1 -> Sum1/2
  Sum1/1 -> Sum2/1

== system smm_with_grf_tilting_2d/Control/Behavior Control/Primary Leg Behavior/Raibert Hopping/Spring Rest Length ==
  Spring Constant : Inport
  Virtual Spring Length [m] : Inport  Port=2
  Measured Leg Force : Inport  Port=3
  Contact [1/0] : Inport  Port=4
  Divide : Product  Inputs=*/
  Hold Initial : Subsystem
  Saturation : Saturate  UpperLimit=inf  LowerLimit=0
  Sum3 : Sum  Inputs=++|
  Rest Length [m] : Outport
  wires:
  Divide/1 -> Sum3/2
  Virtual Spring Length [m]/1 -> Sum3/1
  Measured Leg Force/1 -> Saturation/1
  Sum3/1 -> Hold Initial/1(in)
  Hold Initial/1(out) -> Rest Length [m]/1
  Saturation/1 -> Divide/1
  Contact [1/0]/1 -> Hold Initial/Trigger
  Spring Constant/1 -> Divide/2

== system smm_with_grf_tilting_2d/Control/Behavior Control/Primary Leg Behavior/SMM 01/Primary Stance Phase ==
  note: (alternatively: rotate the GRF vector in the inverse dynamics)
  note: Modulate virtual spring
      | stiffness to regulate
      | energy during stance
  note: Stance
  note: Command a virtual spring
      | force to match the SMM
      | using inverse dynamics
  note: Posture control loop
      | to prevent the torso
      | from falling over
  Primary Leg Length [m m/s] : Inport
  Torso Pitch [rad rad/s] : Inport  Port=2
  Enable Posture Control [1/0] : Inport  Port=3
  Right/Left Primary [1/0] : Inport  Port=4
  System Energy [J] : Inport  Port=5
  Virtual Spring Length [m m/s] : Inport  Port=6
  Primary w [m] : Inport  Port=7
  Primary Leg Angle [rad rad/s] : Inport  Port=8
  E_target1 : Constant  Value=ff_energy_r
  E_target2 : Constant  Value=ff_energy_l
  Nonlinear Spring Stiffness : Subsystem
  Selector3 : Selector  InputPortWidth=2  Indices=[2]
  Sum3 : Sum  Inputs=|+-
  Sum4 : Sum  Inputs=-+|
  Switch1 : Switch  Criteria=u2 ~= 0
  Terminator : Terminator
  Terminator1 : Terminator
  Trunk Balance PD Compensation : Subsystem
  Virtual Leg Force and Swing Leg Retraction : Subsystem
  k_virtual : Gain
  target_energy : Constant  Value=target_energy
  Leg Torque Command [Nm] : Outport
  Leg Force Command [Nm] : Outport  Port=2
  wires:
  Virtual Leg Force and Swing Leg Retraction/2(Leg Torque [Nm]) -> Leg Torque Command [Nm]/1
  Primary Leg Angle [rad rad/s]/1 -> Virtual Leg Force and Swing Leg Retraction/3(Leg Angle [rad rad/s])
  Primary w [m]/1 -> Virtual Leg Force and Swing Leg Retraction/5(Primary w [m])
  Trunk Balance PD Compensation/1(Torque [Nm]) -> Terminator/1
  Virtual Leg Force and Swing Leg Retraction/1(Leg Force [N]) -> Leg Force Command [Nm]/1
  Primary Leg Length [m m/s]/1 -> Virtual Leg Force and Swing Leg Retraction/2(Leg Length [m m/s]), Selector3/1
  Right/Left Primary [1/0]/1 -> Switch1/2
  Torso Pitch [rad rad/s]/1 -> Virtual Leg Force and Swing Leg Retraction/4(Torso Pitch [rad rad/s]), Trunk Balance PD Compensation/1(Torso Pitch [rad rad/s])
  E_target2/1 -> Switch1/3
  Sum4/1 -> Sum3/1
  E_target1/1 -> Switch1/1
  Selector3/1 -> Nonlinear Spring Stiffness/2(dl_virtual [m/s])
  Enable Posture Control [1/0]/1 -> Trunk Balance PD Compensation/Enable
  Sum3/1 -> Nonlinear Spring Stiffness/1(Energy Error [J])
  Nonlinear Spring Stiffness/1(k_virtual [N/m]) -> Virtual Leg Force and Swing Leg Retraction/1(k_virtual [N/m]), k_virtual/1
  Virtual Spring Length [m m/s]/1 -> Virtual Leg Force and Swing Leg Retraction/6(Virtual Spring Length [m m/s])
  target_energy/1 -> Sum4/2
  k_virtual/1 -> Terminator1/1
  System Energy [J]/1 -> Sum3/2
  Switch1/1 -> Sum4/1

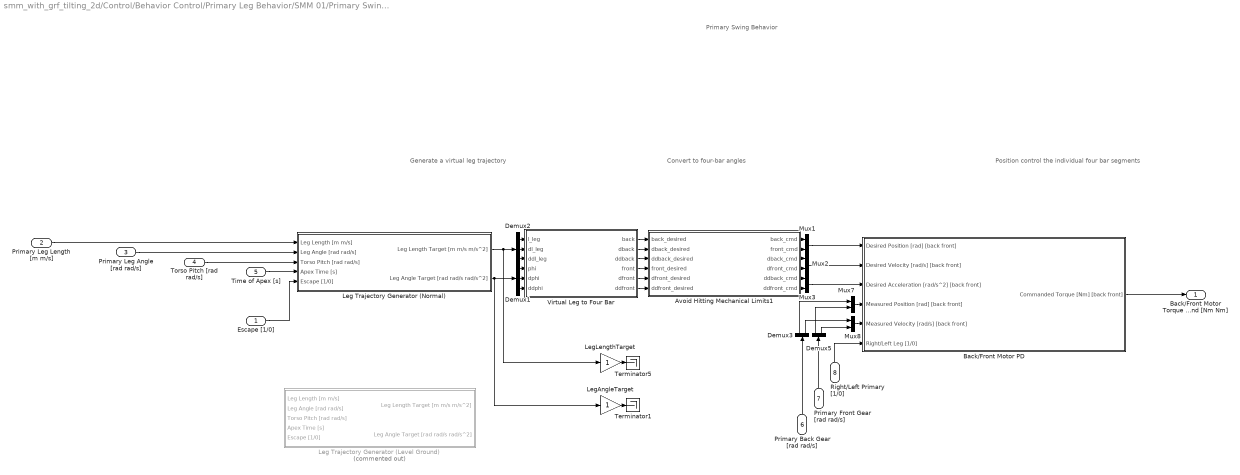
== system smm_with_grf_tilting_2d/Control/Behavior Control/Primary Leg Behavior/SMM 01/Primary Swing Phase ==
  note: Convert to
      | four-bar angles
  note: Primary Swing Behavior
  note: Position control the
      | individual four bar segments
  note: Generate a virtual
      | leg trajectory
  Escape [1/0] : Inport
  Primary Leg Length [m m/s] : Inport  Port=2
  Primary Leg Angle [rad rad/s] : Inport  Port=3
  Torso Pitch [rad rad/s] : Inport  Port=4
  Time of Apex [s] : Inport  Port=5
  Primary Back Gear [rad rad/s] : Inport  Port=6
  Primary Front Gear [rad rad/s] : Inport  Port=7
  Right/Left Primary [1/0] : Inport  Port=8
  Avoid Hitting Mechanical Limits1 : MATLAB Function  TreatAsAtomicUnit=on
  Back/Front Motor PD : Subsystem
  Demux1 : Demux  Outputs=3
  Demux2 : Demux  Outputs=3
  Demux3 : Demux  Outputs=2
  Demux5 : Demux  Outputs=2
  Leg Trajectory Generator (Level Ground) : Subsystem  Commented=on
  Leg Trajectory Generator (Normal) : Subsystem
  LegAngleTarget : Gain
  LegLengthTarget : Gain
  Mux{1..3,7..8} (5 alike) : Mux  Inputs=2
  Terminator1 : Terminator
  Terminator5 : Terminator
  Virtual Leg to Four Bar : MATLAB Function  TreatAsAtomicUnit=on
  Back/Front Motor Torque Command [Nm Nm] : Outport
  wires:
  LegAngleTarget/1 -> Terminator1/1
  Leg Trajectory Generator (Normal)/1(Leg Length Target [m m/s m/s^2]) -> LegLengthTarget/1, Demux2/1
  LegLengthTarget/1 -> Terminator5/1
  Mux3/1 -> Back/Front Motor PD/3(Desired Acceleration [rad/s^2] [back front])
  Mux2/1 -> Back/Front Motor PD/2(Desired Velocity [rad/s] [back front])
  Avoid Hitting Mechanical Limits1/6(ddfront_cmd) -> Mux3/2
  Avoid Hitting Mechanical Limits1/5(ddback_cmd) -> Mux3/1
  Avoid Hitting Mechanical Limits1/4(dfront_cmd) -> Mux2/2
  Avoid Hitting Mechanical Limits1/3(dback_cmd) -> Mux2/1
  Primary Back Gear [rad rad/s]/1 -> Demux3/1
  Primary Front Gear [rad rad/s]/1 -> Demux5/1
  Demux2/1 -> Virtual Leg to Four Bar/1(l_leg)
  Demux1/2 -> Virtual Leg to Four Bar/5(dphi)
  Demux1/1 -> Virtual Leg to Four Bar/4(phi)
  Demux2/2 -> Virtual Leg to Four Bar/2(dl_leg)
  Demux1/3 -> Virtual Leg to Four Bar/6(ddphi)
  Demux2/3 -> Virtual Leg to Four Bar/3(ddl_leg)
  Back/Front Motor PD/1(Commanded Torque [Nm] [back front]) -> Back/Front Motor Torque Command [Nm Nm]/1
  Demux5/1 -> Mux7/2
  Avoid Hitting Mechanical Limits1/1(back_cmd) -> Mux1/1
  Virtual Leg to Four Bar/1(back) -> Avoid Hitting Mechanical Limits1/1(back_desired)
  Avoid Hitting Mechanical Limits1/2(front_cmd) -> Mux1/2
  Virtual Leg to Four Bar/3(ddback) -> Avoid Hitting Mechanical Limits1/3(ddback_desired)
  Virtual Leg to Four Bar/6(ddfront) -> Avoid Hitting Mechanical Limits1/6(ddfront_desired)
  Virtual Leg to Four Bar/4(front) -> Avoid Hitting Mechanical Limits1/4(front_desired)
  Virtual Leg to Four Bar/2(dback) -> Avoid Hitting Mechanical Limits1/2(dback_desired)
  Demux3/1 -> Mux7/1
  Demux3/2 -> Mux8/1
  Torso Pitch [rad rad/s]/1 -> Leg Trajectory Generator (Normal)/3(Torso Pitch [rad rad/s])
  Right/Left Primary [1/0]/1 -> Back/Front Motor PD/6(Right/Left Leg [1/0])
  Primary Leg Angle [rad rad/s]/1 -> Leg Trajectory Generator (Normal)/2(Leg Angle [rad rad/s])
  Primary Leg Length [m m/s]/1 -> Leg Trajectory Generator (Normal)/1(Leg Length [m m/s])
  Mux1/1 -> Back/Front Motor PD/1(Desired Position [rad] [back front])
  Mux7/1 -> Back/Front Motor PD/4(Measured Position [rad] [back front])
  Virtual Leg to Four Bar/5(dfront) -> Avoid Hitting Mechanical Limits1/5(dfront_desired)
  Time of Apex [s]/1 -> Leg Trajectory Generator (Normal)/4(Apex Time [s])
  Demux5/2 -> Mux8/2
  Mux8/1 -> Back/Front Motor PD/5(Measured Velocity [rad/s] [back front])
  Escape [1/0]/1 -> Leg Trajectory Generator (Normal)/5(Escape [1/0])
  Leg Trajectory Generator (Normal)/2(Leg Angle Target [rad rad/s rad/s^2]) -> LegAngleTarget/1, Demux1/1

== system smm_with_grf_tilting_2d/Control/Behavior Control/Secondary Leg Behavior/Back//Front Motor PD/Friction Compensation ==
  Right/Left [1/0] : Inport
  Commanded Velocity [rad/s] [back front] : Inport  Port=2
  Product : Product
  Sign : Signum
  Sum1 : Sum
  Switch : Switch  Criteria=u2 ~= 0
  Switch1 : Switch  Criteria=u2 ~= 0
  coulomb_friction_left : Constant  Value=sea_coulomb_friction(3:4)
  coulomb_friction_right : Constant  Value=sea_coulomb_friction(1:2)
  offset_friction_left : Constant  Value=sea_offset_friction(3:4)
  offset_friction_right : Constant  Value=sea_offset_friction(1:2)
  Friction Compensation [Nm] : Outport
  wires:
  Commanded Velocity [rad/s] [back front]/1 -> Sign/1
  Switch/1 -> Sum1/2
  Sum1/1 -> Friction Compensation [Nm]/1
  Product/1 -> Sum1/1
  Right/Left [1/0]/1 -> Switch1/2, Switch/2
  offset_friction_right/1 -> Switch/1
  offset_friction_left/1 -> Switch/3
  coulomb_friction_right/1 -> Switch1/1
  coulomb_friction_left/1 -> Switch1/3
  Switch1/1 -> Product/2
  Sign/1 -> Product/1

== system smm_with_grf_tilting_2d/Control/Behavior Control/Primary Leg Behavior/Raibert Hopping/Back//Front Motor PD/Friction Compensation ==
  Right/Left [1/0] : Inport
  Commanded Velocity [rad/s] [back front] : Inport  Port=2
  Product : Product
  Sign : Signum
  Sum1 : Sum
  Switch : Switch  Criteria=u2 ~= 0
  Switch1 : Switch  Criteria=u2 ~= 0
  coulomb_friction_left : Constant  Value=sea_coulomb_friction(3:4)
  coulomb_friction_right : Constant  Value=sea_coulomb_friction(1:2)
  offset_friction_left : Constant  Value=sea_offset_friction(3:4)
  offset_friction_right : Constant  Value=sea_offset_friction(1:2)
  Friction Compensation [Nm] : Outport
  wires:
  Commanded Velocity [rad/s] [back front]/1 -> Sign/1
  Switch/1 -> Sum1/2
  Sum1/1 -> Friction Compensation [Nm]/1
  Product/1 -> Sum1/1
  Right/Left [1/0]/1 -> Switch1/2, Switch/2
  offset_friction_right/1 -> Switch/1
  offset_friction_left/1 -> Switch/3
  coulomb_friction_right/1 -> Switch1/1
  coulomb_friction_left/1 -> Switch1/3
  Switch1/1 -> Product/2
  Sign/1 -> Product/1

== system smm_with_grf_tilting_2d/Control/Behavior Control/Primary Leg Behavior/Raibert Hopping/Hold Values/Subsystem ==
  in : Inport
  Enable : EnablePort
  out : Outport  InitialOutput=[0 0 l0_leg l0_leg]
  wires:
  in/1 -> out/1

== system smm_with_grf_tilting_2d/Control/Behavior Control/Primary Leg Behavior/Raibert Hopping/Inverse Dynamics Virtual Spring/Angle Sine Wave ==
  Enable : EnablePort  StatesWhenEnabling=reset  ShowOutputPort=on
  Sine Wave : Sin  TimeSource=Use external signal  Amplitude=torso_wave_amplitude  Frequency=torso_wave_frequency  SampleTime=0
  Timer : Subsystem
  Angle : Outport  OutputWhenDisabled=reset  InitialOutput=[0]
  wires:
  Timer/1(timer [s]) -> Sine Wave/1
  Enable/1 -> Timer/Enable
  Sine Wave/1 -> Angle/1

== system smm_with_grf_tilting_2d/Control/Behavior Control/Primary Leg Behavior/Raibert Hopping/Inverse Dynamics Virtual Spring/Leg Force-Torque Distribution ==
  Front Spring Torque [Nm] : Inport
  Back Spring Torque [Nm] : Inport  Port=2
  w [m] : Inport  Port=3
  Divide : Product  Inputs=*/
  Sum2 : Sum  Inputs=+|+
  Sum5 : Sum  Inputs=+|-
  Leg Force [N] : Outport
  Leg Torque [Nm] : Outport  Port=2
  wires:
  Sum2/1 -> Leg Torque [Nm]/1
  Back Spring Torque [Nm]/1 -> Sum5/2, Sum2/2
  Sum5/1 -> Divide/1
  w [m]/1 -> Divide/2
  Front Spring Torque [Nm]/1 -> Sum5/1, Sum2/1
  Divide/1 -> Leg Force [N]/1

== system smm_with_grf_tilting_2d/Control/Behavior Control/Primary Leg Behavior/Raibert Hopping/Spring Rest Length/Hold Initial ==
  in : Inport
  Trigger : TriggerPort  ShowOutputPort=on  PortDimensions=1
  Subsystem : Subsystem
  out : Outport
  wires:
  Trigger/1 -> Subsystem/Enable
  Subsystem/1(out) -> out/1
  in/1 -> Subsystem/1(in)

== system smm_with_grf_tilting_2d/Control/Behavior Control/Primary Leg Behavior/SMM 01/Primary Stance Phase/Nonlinear Spring Stiffness ==
  Energy Error [J] : Inport
  dl_virtual [m/s] : Inport  Port=2
  Product : Product  Inputs=3
  Saturation : Saturate  UpperLimit=max_k_virtual  LowerLimit=min_k_virtual  ZeroCross=off
  Sum : Sum  Inputs=+|-
  c_energy : Constant  Value=c_energy
  k0_virtual : Constant  Value=k0_virtual
  k_virtual [N/m] : Outport
  wires:
  dl_virtual [m/s]/1 -> Product/2
  c_energy/1 -> Product/3
  k0_virtual/1 -> Sum/1
  Energy Error [J]/1 -> Product/1
  Saturation/1 -> k_virtual [N/m]/1
  Sum/1 -> Saturation/1
  Product/1 -> Sum/2

== system smm_with_grf_tilting_2d/Control/Behavior Control/Primary Leg Behavior/SMM 01/Primary Stance Phase/Trunk Balance PD Compensation ==
  Torso Pitch [rad rad/s] : Inport
  Enable : EnablePort  StatesWhenEnabling=reset
  Constant2 : Constant  Value=0
  Demux : Demux  Outputs=2
  Derivative Gain : Gain  Gain=kd_torso
  Gain1 : Gain  Gain=-1
  Proportional Gain : Gain  Gain=kp_torso
  Reference Lean [rad] : Constant  Value=desired_torso_angle
  Sum1 : Sum  Inputs=|+-
  Sum4 : Sum  Inputs=|+-
  Sum5 : Sum
  Torque [Nm] : Outport  OutputWhenDisabled=reset  InitialOutput=[0]
  wires:
  Sum5/1 -> Gain1/1
  Demux/2 -> Sum1/2
  Constant2/1 -> Sum1/1
  Reference Lean [rad]/1 -> Sum4/1
  Demux/1 -> Sum4/2
  Sum4/1 -> Proportional Gain/1
  Torso Pitch [rad rad/s]/1 -> Demux/1
  Derivative Gain/1 -> Sum5/2
  Proportional Gain/1 -> Sum5/1
  Sum1/1 -> Derivative Gain/1
  Gain1/1 -> Torque [Nm]/1

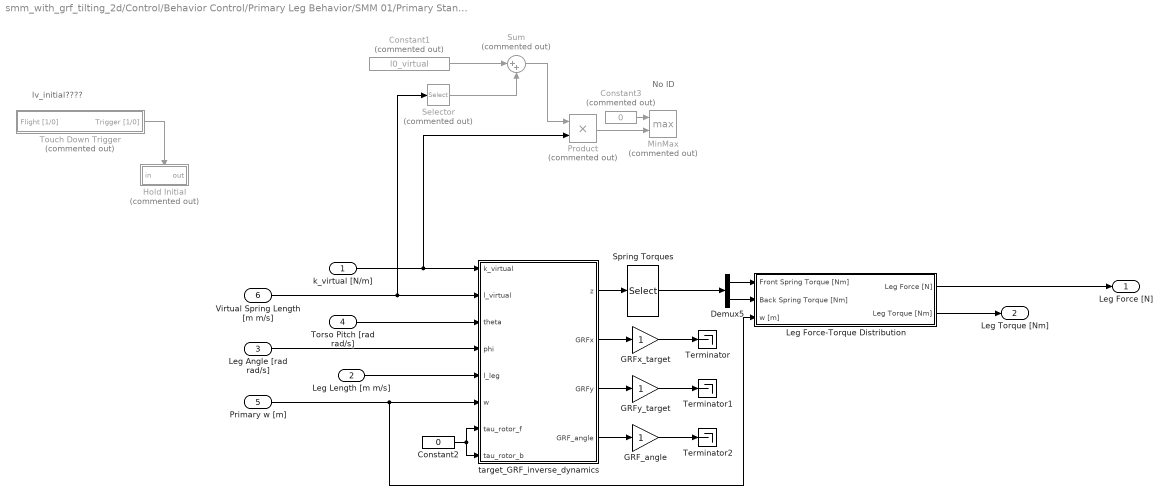
== system smm_with_grf_tilting_2d/Control/Behavior Control/Primary Leg Behavior/SMM 01/Primary Stance Phase/Virtual Leg Force and Swing Leg Retraction ==
  note: lv_initial????
  note: No ID
  k_virtual [N/m] : Inport
  Leg Length [m m/s] : Inport  Port=2
  Leg Angle [rad rad/s] : Inport  Port=3
  Torso Pitch [rad rad/s] : Inport  Port=4
  Primary w [m] : Inport  Port=5
  Virtual Spring Length [m m/s] : Inport  Port=6
  Constant1 : Constant  Commented=on  Value=l0_virtual
  Constant2 : Constant  Value=0
  Constant3 : Constant  Commented=on  Value=0
  Demux5 : Demux  Outputs=2
  GRF_angle : Gain
  GRFx_target : Gain
  GRFy_target : Gain
  Hold Initial : Subsystem  Commented=on
  Leg Force-Torque Distribution : Subsystem
  MinMax : MinMax  Commented=on  Function=max  Inputs=2
  Product : Product  Commented=on
  Selector : Selector  Commented=on  InputPortWidth=2  Indices=[1]
  Spring Torques : Selector  InputPortWidth=7  Indices=[6 7]
  Sum : Sum  Commented=on  Inputs=|++
  Terminator : Terminator
  Terminator1 : Terminator
  Terminator2 : Terminator
  Touch Down Trigger : Subsystem  Commented=on
  target_GRF_inverse_dynamics : MATLAB Function  TreatAsAtomicUnit=on
  Leg Force [N] : Outport
  Leg Torque [Nm] : Outport  Port=2
  wires:
  Leg Force-Torque Distribution/1(Leg Force [N]) -> Leg Force [N]/1
  Constant3/1 -> MinMax/1
  Product/1 -> MinMax/2
  Sum/1 -> Product/1
  Selector/1 -> Sum/2
  Constant1/1 -> Sum/1
  GRF_angle/1 -> Terminator2/1
  GRFy_target/1 -> Terminator1/1
  GRFx_target/1 -> Terminator/1
  Leg Angle [rad rad/s]/1 -> target_GRF_inverse_dynamics/4(phi)
  Torso Pitch [rad rad/s]/1 -> target_GRF_inverse_dynamics/3(theta)
  target_GRF_inverse_dynamics/4(GRF_angle) -> GRF_angle/1
  target_GRF_inverse_dynamics/3(GRFy) -> GRFy_target/1
  target_GRF_inverse_dynamics/2(GRFx) -> GRFx_target/1
  Leg Force-Torque Distribution/2(Leg Torque [Nm]) -> Leg Torque [Nm]/1
  Primary w [m]/1 -> target_GRF_inverse_dynamics/6(w), Leg Force-Torque Distribution/3(w [m])
  Spring Torques/1 -> Demux5/1
  Demux5/1 -> Leg Force-Torque Distribution/1(Front Spring Torque [Nm])
  Demux5/2 -> Leg Force-Torque Distribution/2(Back Spring Torque [Nm])
  target_GRF_inverse_dynamics/1(z) -> Spring Torques/1
  Constant2/1 -> target_GRF_inverse_dynamics/8(tau_rotor_b), target_GRF_inverse_dynamics/7(tau_rotor_f)
  Leg Length [m m/s]/1 -> target_GRF_inverse_dynamics/5(l_leg)
  Touch Down Trigger/1(Trigger [1/0]) -> Hold Initial/Trigger
  k_virtual [N/m]/1 -> target_GRF_inverse_dynamics/1(k_virtual), Product/2
  Virtual Spring Length [m m/s]/1 -> target_GRF_inverse_dynamics/2(l_virtual), Selector/1
